simulink model "rotpentemplate2"  (R2021b)
settings: Solver=ode45  StartTime=0.0  StopTime=TSim  RelTol=1e-3  EnableMultiTasking=on
values from neighbouring files (symbols this model uses):
  h = 0.01    [MPC.m]    (also in MPC_poly.m = 0.05; Robus_controller.m; data_ext.m = 0.05)
undefined symbols (not defined in the file or in its folder): adingain, adinoffs, daoutgain, daoutoffs
settings Model: Creator=rbabuska  LastModifiedBy=jmarcar
settings SolverCC: AlgebraicLoopSolver=TrustRegion
settings DataIOCC: LimitDataPoints=on  SaveFormat=Array  ReturnWorkspaceOutputs=off  SignalLoggingName=sigsOut
settings OptimizationCC: BooleanDataType=off  ExpressionDepthLimit=2147483647  InitFltsAndDblsToZero=on  LifeSpan=inf
settings DebuggingCC: SaveWithParameterizedLinksMsg=none  SignalResolutionControl=TryResolveAllWithWarning  MultiTaskDSMMsg=warning  MultiTaskCondExecSysMsg=none  AllowSymbolicDim=off  StateNameClashWarn=warning  SFUnexpectedBacktrackingDiag=warning  SFNoUnconditionalDefaultTransitionDiag=warning  SFExecutionAtInitializationDiag=none  SFMachineParentedDataDiag=warning  ArithmeticOperatorsInVariantConditions=warning
settings HardwareCC: ProdBitPerPointer=32  ProdBitPerSizeT=32  ProdBitPerPtrDiffT=32  ProdLargestAtomicFloat=None  ProdIntDivRoundTo=Undefined  ProdEndianess=Unspecified  ProdWordSize=32  ProdHWDeviceType=32-bit Generic  TargetUnknown=on
settings ModelReferenceCC: PropagateSignalLabelsOutOfModel=off
settings SFSimCC: SimUseLocalCustomCode=off  CustomCodeUndefinedFunction=UseInterfaceOnly
settings RTWCC: RTWUseLocalCustomCode=off
settings CodeAppCC: StateflowObjectComments=on
settings GRTTargetCC: TargetFcnLib=ansi_tfl_tmw.mat  TargetLangStandard=C89/C90 (ANSI)  CombineOutputUpdateFcns=off  GRTInterface=on
settings ConfigComp: CovMetricSettings=dw  CovSaveCumulativeToWorkspaceVar=on  CovSaveSingleToWorkspaceVar=on  CovExternalEMLEnable=off

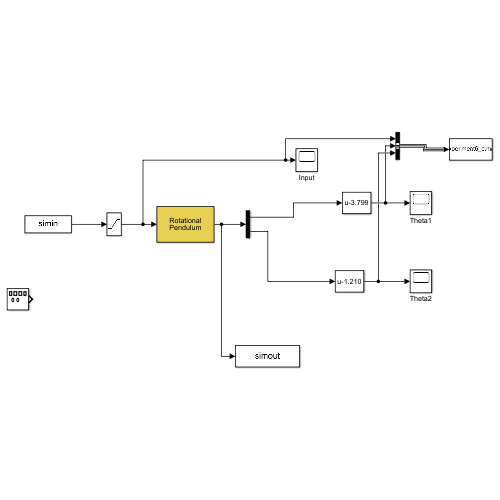
[thumbnail: Simulink's stored preview of the top-level diagram]
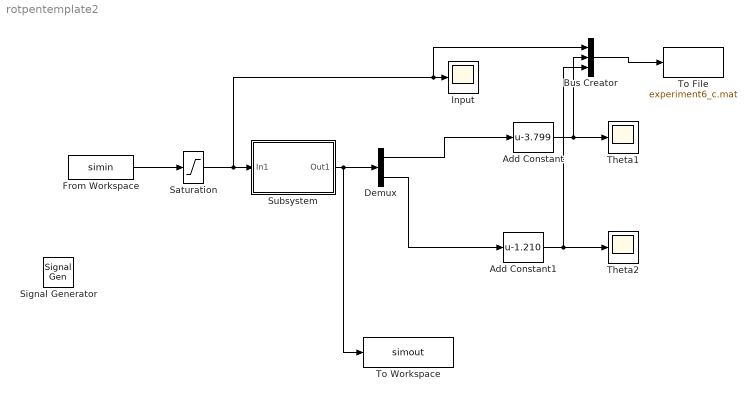
== system rotpentemplate2 ==
  Add Constant : Bias  Bias=-3.799
  Add Constant1 : Bias  Bias=-1.210
  Bus Creator : BusCreator  Inputs=3
  Demux : Demux  Outputs=2
  From Workspace : FromWorkspace  VariableName=simin
  Input : Scope
  Saturation : Saturate  UpperLimit=1  LowerLimit=-1
  Signal Generator : SignalGenerator  Amplitude=0.1
  Subsystem : Subsystem
      mask Display: disp('Rotational\nPendulum')
  Theta1 : Scope
  Theta2 : Scope
  To File : ToFile  Filename=experiment6_c.mat
  To Workspace : ToWorkspace  VariableName=simout  SaveFormat=Timeseries  SampleTime=-1
  wires:
  Saturation/1 -> Subsystem/1(In1), Bus Creator/1, Input/1
  Subsystem/1(Out1) -> To Workspace/1, Demux/1
  Demux/1 -> Add Constant/1
  Demux/2 -> Add Constant1/1
  From Workspace/1 -> Saturation/1
  Add Constant/1 -> Bus Creator/2, Theta1/1
  Add Constant1/1 -> Theta2/1, Bus Creator/3
  Bus Creator/1 -> To File/1

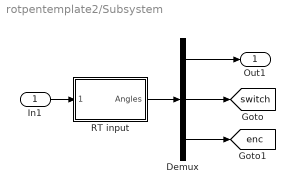
== system rotpentemplate2/Subsystem ==
  In1 : Inport
  Demux : Demux  Outputs=[2 4 1]
  RT input : Subsystem  mask{Ts=h, channels=[6 7]}
      mask prompts: Ts "Sample time [s]:"; channels "Channels to read (e.g., [6 7])"
      mask init:
      | hwinit;
      | 
      | % initialize FPGA
      | fugihandle = fugiboard('Open', 'Pendulum1');
      | fugihandle.WatchdogTimeout = 0.5;
      | fugiboard('SetParams', fugihandle);
      | fugiboard('Write', fugihandle, 0, 0, 0, 0);  % dummy write to sync interface board
      | fugiboard('Write', fugihandle, 5, 1, 0, 0);  % reset position, activate relay
      | data = fugiboard('Read', fugihandle);        % get version info from FPGA
      | % model = bitshift(data(1), -5); 
      | % version = bitand(data(1), 31);
      | % disp(sprintf('FPGA setup %d, version %d', model, version)); % for the B&P it should say 1 1, or else there is a problem
      | fugiboard('Write', fugihandle, 0, 1, 0, 0);  % end reset
      | pause(0.1);                         % give relay some time to respond
      mask Display: disp('Rotational\nPendulum')
  Out1 : Outport
  tag scope: enc=global, switch=global
  wires:
  RT input/1(Angles) -> Demux/1
  Demux/1 -> Out1/1
  Demux/2 -> [switch]
  Demux/3 -> [enc]
  In1/1 -> RT input/1(Motors)

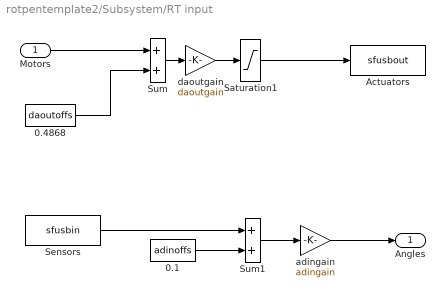
== system rotpentemplate2/Subsystem/RT input ==
  Motors : Inport
  0.1 : Constant  Value=adinoffs
  0.4868 : Constant  Value=daoutoffs
  Actuators : S-Function  FunctionName=sfusbout  Parameters=Ts, fugihandle  SFunctionDeploymentMode=off  EnableBusSupport=off
  Saturation1 : Saturate  UpperLimit=10  LowerLimit=-10
  Sensors : S-Function  FunctionName=sfusbin  Parameters=Ts, fugihandle, channels  SFunctionDeploymentMode=off  EnableBusSupport=off
  Sum : Sum  InputSameDT=on  SaturateOnIntegerOverflow=on  OutDataTypeStr=Inherit: Same as first input
  Sum1 : Sum  InputSameDT=on  SaturateOnIntegerOverflow=on  OutDataTypeStr=Inherit: Same as first input
  adingain : Gain  Gain=adingain  SaturateOnIntegerOverflow=on  OutDataTypeStr=Inherit: Same as input  ParamDataTypeStr=Inherit: Same as input
  daoutgain : Gain  Gain=daoutgain  SaturateOnIntegerOverflow=on  OutDataTypeStr=Inherit: Same as input  ParamDataTypeStr=Inherit: Same as input
  Angles : Outport
  wires:
  Sum/1 -> daoutgain/1
  0.4868/1 -> Sum/2
  Motors/1 -> Sum/1
  Sum1/1 -> adingain/1
  0.1/1 -> Sum1/2
  adingain/1 -> Angles/1
  Saturation1/1 -> Actuators/1
  daoutgain/1 -> Saturation1/1
  Sensors/1 -> Sum1/1
